simulink subsystem "PvtSubSys_LATC"  (R2020b)
settings: Solver=VariableStepAuto  StartTime=0.0  StopTime=10.0  RelTol=1e-3
values from neighbouring files (symbols this model uses):
  P_Global_CharSpd_ms : value not decoded    [PubParsGlobal.sldd]
  P_Global_SteeringAngleRatio : value not decoded    [PubParsGlobal.sldd]
  P_Global_WheelBase_m : value not decoded    [PubParsGlobal.sldd]
  P_LCS_A0_Dis_BP : value not decoded    [SubMdlDD_LATC.sldd]
  P_LCS_A2_Curve_BP : value not decoded    [SubMdlDD_LATC.sldd]
  P_LCS_A2_LatAcc_BP : value not decoded    [SubMdlDD_LATC.sldd]
  P_LCS_A2_Pretime = 0.075    [SubMdlDD_LATC.sldd]
  P_LCS_A2S_FliterTime = 0.5    [SubMdlDD_LATC.sldd]
  P_LCS_AngErrReversSign_SourceSW = 1.0    [SubMdlDD_LATC.sldd]
  P_LCS_AngleErrorReversTorq : value not decoded    [SubMdlDD_LATC.sldd]
  P_LCS_AngleErrorReversTorq_LC_TarAngleBp : value not decoded    [SubMdlDD_LATC.sldd]
  P_LCS_AngleErrorReversTorq_LC_TarAngleFac : value not decoded    [SubMdlDD_LATC.sldd]
  P_LCS_AngleErrorReversTorq_LC_VehSpdBp : value not decoded    [SubMdlDD_LATC.sldd]
  P_LCS_AngleErrorReversTorq_LC_VehSpdVal : value not decoded    [SubMdlDD_LATC.sldd]
  P_LCS_AngleErrorReversTorq_VehSpdBp : value not decoded    [SubMdlDD_LATC.sldd]
  P_LCS_AngleErrorReversTorq_VehSpdFac : value not decoded    [SubMdlDD_LATC.sldd]
  P_LCS_AngleFilterTime = 0.1    [SubMdlDD_LATC.sldd]
  P_LCS_AngleSlope_AES_Active = 0.4 0.4 0.4 0.35 0.35 0.35 0.35 0.35 0.35 0.3 0.3 0.3 0.3 0.3 0.3 0.3 0.3 0.3 0.3 0.4 0.4 0.4 0.35 0.35 0.35 0.35 0.35 0.35 0.3 0.3 0.3 0.3 0.3 0.3 0.3 0.3 0.3 0.3 0.4 0.4 0.4 0.35 0.35 0.35 0.35 0.35 0.35 0.3 0.3 0.3 0.3 0.3 0.3 0.3 0.3 0.3 0.3 0.4 0.4 0.4 0.35 0.35 0.35 0.35 0.35 0.35 0.3 0.3 0.3 0.3 0.3 0.3 0.3 0.3 0.3 0.3 0.4 0.4 0.4 0.35 0.35 0.35 0.35 0.35 0.35 0.3 0.3 0.3 0.3 0.3 0.3 0.3 0.    [SubMdlDD_LATC.sldd]
  P_LCS_AngleSlope_ESS_Add = 1.0 1.0 1.0 1.0 2.0 2.0 2.0 7.0 7.0 7.0 7.0 7.0 7.0 7.0 7.0 7.0 7.0 7.0 7.0 1.0 1.0 1.0 1.0 2.0 2.0 2.0 7.0 7.0 7.0 7.0 7.0 7.0 7.0 7.0 7.0 7.0 7.0 7.0 1.0 1.0 1.0 1.0 2.0 2.0 2.0 7.0 7.0 7.0 7.0 7.0 7.0 7.0 7.0 7.0 7.0 7.0 7.0 1.0 1.0 1.0 1.0 2.0 2.0 2.0 7.0 7.0 7.0 7.0 7.0 7.0 7.0 7.0 7.0 7.0 7.0 7.0 1.0 1.0 1.0 1.0 7.5 7.5 7.5 7.5 7.5 7.5 7.5 7.5 7.5 7.5 7.5 8.0 8.0 8.0 8.0 1.0 1.0 1.0 1.0 7.5    [SubMdlDD_LATC.sldd]
  P_LCS_AngleSlope_LC_Eco = 0.4 0.4 0.4 0.35 0.35 0.35 0.35 0.35 0.35 0.3 0.3 0.3 0.3 0.3 0.3 0.3 0.3 0.3 0.3 0.4 0.4 0.4 0.35 0.35 0.35 0.35 0.35 0.35 0.3 0.3 0.3 0.3 0.3 0.3 0.3 0.3 0.3 0.3 0.4 0.4 0.4 0.35 0.35 0.35 0.35 0.35 0.35 0.3 0.3 0.3 0.3 0.3 0.3 0.3 0.3 0.3 0.3 0.4 0.4 0.4 0.35 0.35 0.35 0.35 0.35 0.35 0.3 0.3 0.3 0.3 0.3 0.3 0.3 0.3 0.3 0.3 0.4 0.4 0.4 0.35 0.35 0.35 0.35 0.35 0.35 0.3 0.3 0.3 0.3 0.3 0.3 0.3 0.    [SubMdlDD_LATC.sldd]
  P_LCS_AngleSlope_LC_Nomal = 0.4 0.4 0.4 0.35 0.35 0.35 0.35 0.35 0.35 0.3 0.3 0.3 0.3 0.3 0.3 0.3 0.3 0.3 0.3 0.4 0.4 0.4 0.35 0.35 0.35 0.35 0.35 0.35 0.3 0.3 0.3 0.3 0.3 0.3 0.3 0.3 0.3 0.3 0.4 0.4 0.4 0.35 0.35 0.35 0.35 0.35 0.35 0.3 0.3 0.3 0.3 0.3 0.3 0.3 0.3 0.3 0.3 0.4 0.4 0.4 0.35 0.35 0.35 0.35 0.35 0.35 0.3 0.3 0.3 0.3 0.3 0.3 0.3 0.3 0.3 0.3 0.4 0.4 0.4 0.35 0.35 0.35 0.35 0.35 0.35 0.3 0.3 0.3 0.3 0.3 0.3 0.3 0.    [SubMdlDD_LATC.sldd]
  P_LCS_AngleSlope_LC_Sport = 0.4 0.4 0.4 0.35 0.35 0.35 0.35 0.35 0.35 0.3 0.3 0.3 0.3 0.3 0.3 0.3 0.3 0.3 0.3 0.4 0.4 0.4 0.35 0.35 0.35 0.35 0.35 0.35 0.3 0.3 0.3 0.3 0.3 0.3 0.3 0.3 0.3 0.3 0.4 0.4 0.4 0.35 0.35 0.35 0.35 0.35 0.35 0.3 0.3 0.3 0.3 0.3 0.3 0.3 0.3 0.3 0.3 0.4 0.4 0.4 0.35 0.35 0.35 0.35 0.35 0.35 0.3 0.3 0.3 0.3 0.3 0.3 0.3 0.3 0.3 0.3 0.4 0.4 0.4 0.35 0.35 0.35 0.35 0.35 0.35 0.3 0.3 0.3 0.3 0.3 0.3 0.3 0.    [SubMdlDD_LATC.sldd]
  P_LCS_AngleSlope_LCK = 0.4 0.4 0.4 0.4 0.4 0.4 0.4 0.4 0.4 0.4 0.4 0.4 0.4 0.4 0.4 0.4 0.4 0.4 0.4 0.4 0.4 0.4 0.4 0.4 0.4 0.4 0.4 0.4 0.4 0.4 0.4 0.4 0.4 0.4 0.4 0.4 0.4 0.4 0.4 0.4 0.4 0.4 0.4 0.4 0.4 0.4 0.4 0.4 0.4 0.4 0.4 0.4 0.4 0.4 0.4 0.4 0.4 0.4 0.4 0.4 0.4 0.4 0.4 0.4 0.4 0.4 0.4 0.4 0.4 0.4 0.4 0.4 0.4 0.4 0.4 0.4 0.4 0.4 0.4 0.4 0.4 0.4 0.4 0.4 0.4 0.4 0.4 0.4 0.4 0.4 0.4 0.4 0.4 0.4 0.4 0.4 0.4 0.4 0.4 0.4    [SubMdlDD_LATC.sldd]
  P_LCS_AngleSlope_LCKIE = 0.4 0.4 0.4 0.4 0.4 0.4 0.4 0.4 0.4 0.4 0.4 0.4 0.4 0.4 0.4 0.4 0.4 0.4 0.4 0.4 0.4 0.4 0.4 0.4 0.4 0.4 0.4 0.4 0.4 0.4 0.4 0.4 0.4 0.4 0.4 0.4 0.4 0.4 0.4 0.4 0.4 0.4 0.4 0.4 0.4 0.4 0.4 0.4 0.4 0.4 0.4 0.4 0.4 0.4 0.4 0.4 0.4 0.4 0.4 0.4 0.4 0.4 0.4 0.4 0.4 0.4 0.4 0.4 0.4 0.4 0.4 0.4 0.4 0.4 0.4 0.4 0.4 0.4 0.4 0.4 0.4 0.4 0.4 0.4 0.4 0.4 0.4 0.4 0.4 0.4 0.4 0.4 0.4 0.4 0.4 0.4 0.4 0.4 0.4 0.4    [SubMdlDD_LATC.sldd]
  P_LCS_AngleSlope_LKA = 0.2 0.2 0.3 0.4 0.4 0.4 0.4 0.4 0.4 0.4 0.4 0.4 0.4 0.4 0.4 0.4 0.4 0.4 0.4 0.2 0.2 0.3 0.4 0.4 0.4 0.4 0.4 0.4 0.4 0.4 0.4 0.4 0.4 0.4 0.4 0.4 0.4 0.4 0.2 0.2 0.3 0.4 0.4 0.4 0.4 0.4 0.4 0.4 0.4 0.4 0.4 0.4 0.4 0.4 0.4 0.4 0.4 0.2 0.2 0.3 0.4 0.4 0.4 0.4 0.4 0.4 0.4 0.4 0.4 0.4 0.4 0.4 0.4 0.4 0.4 0.4 0.2 0.2 0.3 0.4 0.4 0.4 0.4 0.4 0.4 0.4 0.4 0.4 0.4 0.4 0.4 0.4 0.4 0.4 0.4 0.2 0.2 0.3 0.4 0.4    [SubMdlDD_LATC.sldd]
  P_LCS_AngleSlope_Spd_BP : value not decoded    [SubMdlDD_LATC.sldd]
  P_LCS_CurAngleFiltEnable = 1    [SubMdlDD_LATC.sldd]
  P_LCS_CurAngleFilterFC = 2.0    [SubMdlDD_LATC.sldd]
  P_LCS_CurentOffset_LimitValue = 0.001    [SubMdlDD_LATC.sldd]
  P_LCS_CurOffset_SterAngleSpd_Enable = 0.0    [SubMdlDD_LATC.sldd]
  P_LCS_CurOffset_SterAngleSpd_LimitValue = 6.0    [SubMdlDD_LATC.sldd]
  P_LCS_CurOffset_VehicleSpd_LimitValue = 7.0    [SubMdlDD_LATC.sldd]
  P_LCS_CurOffsetA2_Enable = 0.0    [SubMdlDD_LATC.sldd]
  P_LCS_CurOffsetA2_FliterTime = 0.2    [SubMdlDD_LATC.sldd]
  P_LCS_DeltaEps_SpdBp : value not decoded    [SubMdlDD_LATC.sldd]
  P_LCS_DeltaEps_TimeVal : value not decoded    [SubMdlDD_LATC.sldd]
  P_LCS_DesAngle_DelaySample : value not decoded    [SubMdlDD_LATC.sldd]
  P_LCS_DetNoOverRide_DrvTrq_TH : value not decoded    [SubMdlDD_LATC.sldd]
  P_LCS_DetOverRide_DrvTrq_TH : value not decoded    [SubMdlDD_LATC.sldd]
  P_LCS_EPSNotActiveSpdValue = 3.0    [SubMdlDD_LATC.sldd]
  P_LCS_ESS_AngleSlope_Limit = 2.9    [SubMdlDD_LATC.sldd]
  P_LCS_ESS_LogicTest_Enable = 1.0    [SubMdlDD_LATC.sldd]
  P_LCS_ESS_MaxTorqSlope : value not decoded    [SubMdlDD_LATC.sldd]
  P_LCS_ESS_NotActiveFlgDelayTime = 0.0    [SubMdlDD_LATC.sldd]
  P_LCS_ESS_NotActiveFlgDelayTimeSW = 0.0    [SubMdlDD_LATC.sldd]
  P_LCS_ESS_SteerAngleErr : value not decoded    [SubMdlDD_LATC.sldd]
  P_LCS_ESS_SteerAngleFilterTime = 0.2    [SubMdlDD_LATC.sldd]
  P_LCS_ESS_TarAngleFilterTime = 0.2    [SubMdlDD_LATC.sldd]
  P_LCS_ESSAngleSW2 = 0.0    [SubMdlDD_LATC.sldd]
  P_LCS_ESSOverrideTime1 = 0.06    [SubMdlDD_LATC.sldd]
  P_LCS_ESSOverrideTime2 = 0.06    [SubMdlDD_LATC.sldd]
  P_LCS_ESSOverrideTime3 = 0.06    [SubMdlDD_LATC.sldd]
  P_LCS_ESSOverrideValue1 = 20.0    [SubMdlDD_LATC.sldd]
  P_LCS_ESSOverrideValue2 = 20.0    [SubMdlDD_LATC.sldd]
  P_LCS_FF_A0_Speed_Factor : value not decoded    [SubMdlDD_LATC.sldd]
  P_LCS_FF_A0_Torq : value not decoded    [SubMdlDD_LATC.sldd]
  P_LCS_FF_EnableSpd = 5.0    [SubMdlDD_LATC.sldd]
  P_LCS_FF_LCRevs_SpdBP : value not decoded    [SubMdlDD_LATC.sldd]
  P_LCS_FF_LCRevs_SpdVal : value not decoded    [SubMdlDD_LATC.sldd]
  P_LCS_FF_LCRevs_TimeBP : value not decoded    [SubMdlDD_LATC.sldd]
  P_LCS_FF_LCRevs_TimeFacVal : value not decoded    [SubMdlDD_LATC.sldd]
  P_LCS_FF_Param_CurveBp : value not decoded    [SubMdlDD_LATC.sldd]
  P_LCS_FF_Param_CurveFac : value not decoded    [SubMdlDD_LATC.sldd]
  P_LCS_FF_Speed_Bp : value not decoded    [SubMdlDD_LATC.sldd]
  P_LCS_FF_Speed_Factor : value not decoded    [SubMdlDD_LATC.sldd]
  P_LCS_FF_TarAngleTorq_Bp : value not decoded    [SubMdlDD_LATC.sldd]
  P_LCS_FF_TarAngleTorq_Factor : value not decoded    [SubMdlDD_LATC.sldd]
  P_LCS_FFW_Torq_AngleBp : value not decoded    [SubMdlDD_LATC.sldd]
  P_LCS_FFW_Torq_SpdBp : value not decoded    [SubMdlDD_LATC.sldd]
  P_LCS_FFW_Torq_V71 : value not decoded    [SubMdlDD_LATC.sldd]
  P_LCS_FFWSwitch : value not decoded    [SubMdlDD_LATC.sldd]
  P_LCS_IN_Offset_Test_SW = 0.0    [SubMdlDD_LATC.sldd]
  P_LCS_IN_Offset_Test_Value = 0.0    [SubMdlDD_LATC.sldd]
  P_LCS_LatAcc2CurveSW = 0.0    [SubMdlDD_LATC.sldd]
  P_LCS_LC_Complete_PreDisFac : value not decoded    [SubMdlDD_LATC.sldd]
  P_LCS_LCK_preDis_Nomal : value not decoded    [SubMdlDD_LATC.sldd]
  P_LCS_MaxTorqSlope : value not decoded    [SubMdlDD_LATC.sldd]
  P_LCS_NoOverRideTime_TH_s : value not decoded    [SubMdlDD_LATC.sldd]
  P_LCS_Offset_FliterTime = 2.0    [SubMdlDD_LATC.sldd]
  P_LCS_OverRideDetect_enable : value not decoded    [SubMdlDD_LATC.sldd]
  P_LCS_OverRideTime_TH_s : value not decoded    [SubMdlDD_LATC.sldd]
  P_LCS_PID_A0_BP : value not decoded    [SubMdlDD_LATC.sldd]
  P_LCS_PID_A0_FF_SW = 0.0    [SubMdlDD_LATC.sldd]
  P_LCS_PID_A0_P : value not decoded    [SubMdlDD_LATC.sldd]
  P_LCS_PID_AngErrFacBp : value not decoded    [SubMdlDD_LATC.sldd]
  P_LCS_PID_AngErrFacBp_P : value not decoded    [SubMdlDD_LATC.sldd]
  P_LCS_PID_AngErrFacVal : value not decoded    [SubMdlDD_LATC.sldd]
  P_LCS_PID_AngErrFacVal_P : value not decoded    [SubMdlDD_LATC.sldd]
  P_LCS_PID_DisableKi_CurveVal = 0.003    [SubMdlDD_LATC.sldd]
  P_LCS_PID_DrvTorqFacBp : value not decoded    [SubMdlDD_LATC.sldd]
  P_LCS_PID_DrvTorqFacVal : value not decoded    [SubMdlDD_LATC.sldd]
  P_LCS_PID_Ki_TarAng_ESS : value not decoded    [SubMdlDD_LATC.sldd]
  P_LCS_PID_Kp_TarAng_ESS : value not decoded    [SubMdlDD_LATC.sldd]
  P_LCS_PID_Kp_TarAng_ESS2 : value not decoded    [SubMdlDD_LATC.sldd]
  P_LCS_PID_Kp_TarTorq_ESS : value not decoded    [SubMdlDD_LATC.sldd]
  P_LCS_PID_Param_CurveBp : value not decoded    [SubMdlDD_LATC.sldd]
  P_LCS_PID_Param_CurveFac : value not decoded    [SubMdlDD_LATC.sldd]
  P_LCS_PID_Param_GainSwitch : value not decoded    [SubMdlDD_LATC.sldd]
  P_LCS_PID_Param_Kd : value not decoded    [SubMdlDD_LATC.sldd]
  P_LCS_PID_Param_KdFilterTime : value not decoded    [SubMdlDD_LATC.sldd]
  P_LCS_PID_Param_Ki : value not decoded    [SubMdlDD_LATC.sldd]
  P_LCS_PID_Param_KiFreaseWhenLC_Enable : value not decoded    [SubMdlDD_LATC.sldd]
  P_LCS_PID_Param_Kp : value not decoded    [SubMdlDD_LATC.sldd]
  P_LCS_PID_Param_Speed_Adapt : value not decoded    [SubMdlDD_LATC.sldd]
  P_LCS_PID_Param_Speed_Factor_D : value not decoded    [SubMdlDD_LATC.sldd]
  P_LCS_PID_Param_Speed_Factor_I : value not decoded    [SubMdlDD_LATC.sldd]
  P_LCS_PID_Param_Speed_Factor_P : value not decoded    [SubMdlDD_LATC.sldd]
  P_LCS_PID_Param_SteerWheelAngle_Adapt : value not decoded    [SubMdlDD_LATC.sldd]
  P_LCS_PID_Param_SteerWheelAngle_Factor_D : value not decoded    [SubMdlDD_LATC.sldd]
  P_LCS_PID_Param_SteerWheelAngle_Factor_P : value not decoded    [SubMdlDD_LATC.sldd]
  P_LCS_PID_Param_SteerWheelSpd_Adapt : value not decoded    [SubMdlDD_LATC.sldd]
  P_LCS_PID_Param_SteerWheelSpd_Factor_D : value not decoded    [SubMdlDD_LATC.sldd]
  P_LCS_PID_Param_SteerWheelSpd_Factor_P : value not decoded    [SubMdlDD_LATC.sldd]
  P_LCS_PID_SteerAngSpdLim : value not decoded    [SubMdlDD_LATC.sldd]
  P_LCS_preDis_AES_Fac = 0.0 0.0 0.0 0.0 -0.1 -0.1 -0.1 -0.1 -0.1 -0.1 0.1 0.1 0.1 0.2 0.2 0.2 0.2 0.2 0.2 0.0 0.0 0.0 0.0 -0.1 -0.1 -0.1 -0.1 -0.1 -0.1 0.1 0.1 0.1 0.2 0.2 0.2 0.2 0.2 0.2 0.0 0.0 0.0 0.0 -0.1 -0.1 -0.1 -0.1 -0.1 -0.1 0.1 0.1 0.1 0.2 0.2 0.2 0.2 0.2 0.2 0.0 0.0 0.0 0.0 -0.1 -0.1 -0.1 -0.1 -0.1 -0.1 0.1 0.1 0.1 0.2 0.2 0.2 0.2 0.2 0.2 0.0 0.0 0.0 0.0 -0.1 -0.1 -0.1 -0.1 -0.1 -0.1 0.2 0.2 0.2 0.35 0.35 0.35    [SubMdlDD_LATC.sldd]
  P_LCS_preDis_LC_Eco_Fac = 0.0 0.0 0.0 0.0 0.25 0.3 0.3 0.3 0.35 0.35 0.45 0.45 0.45 0.55 0.55 0.55 0.55 0.55 0.55 0.0 0.0 0.0 0.0 0.25 0.3 0.3 0.3 0.35 0.35 0.45 0.45 0.45 0.55 0.55 0.55 0.55 0.55 0.55 0.0 0.0 0.0 0.0 0.25 0.3 0.3 0.3 0.35 0.35 0.45 0.45 0.45 0.55 0.55 0.55 0.55 0.55 0.55 0.0 0.0 0.0 0.0 0.25 0.3 0.3 0.3 0.35 0.35 0.45 0.45 0.45 0.55 0.55 0.55 0.55 0.55 0.55 0.0 0.0 0.0 0.0 0.25 0.3 0.3 0.3 0.35 0.35 0.55    [SubMdlDD_LATC.sldd]
  P_LCS_preDis_LC_Fac = 0.0 0.0 0.0 0.0 -0.1 -0.1 -0.1 -0.1 -0.1 -0.1 0.1 0.1 0.1 0.2 0.2 0.2 0.2 0.2 0.2 0.0 0.0 0.0 0.0 -0.1 -0.1 -0.1 -0.1 -0.1 -0.1 0.1 0.1 0.1 0.2 0.2 0.2 0.2 0.2 0.2 0.0 0.0 0.0 0.0 -0.1 -0.1 -0.1 -0.1 -0.1 -0.1 0.1 0.1 0.1 0.2 0.2 0.2 0.2 0.2 0.2 0.0 0.0 0.0 0.0 -0.1 -0.1 -0.1 -0.1 -0.1 -0.1 0.1 0.1 0.1 0.2 0.2 0.2 0.2 0.2 0.2 0.0 0.0 0.0 0.0 -0.1 -0.1 -0.1 -0.1 -0.1 -0.1 0.2 0.2 0.2 0.35 0.35 0.35    [SubMdlDD_LATC.sldd]
  P_LCS_preDis_LC_Nomal_Fac = 0.0 0.0 0.0 0.0 -0.1 -0.1 -0.1 -0.1 -0.1 -0.1 0.1 0.1 0.1 0.2 0.2 0.2 0.2 0.2 0.2 0.0 0.0 0.0 0.0 -0.1 -0.1 -0.1 -0.1 -0.1 -0.1 0.1 0.1 0.1 0.2 0.2 0.2 0.2 0.2 0.2 0.0 0.0 0.0 0.0 -0.1 -0.1 -0.1 -0.1 -0.1 -0.1 0.1 0.1 0.1 0.2 0.2 0.2 0.2 0.2 0.2 0.0 0.0 0.0 0.0 -0.1 -0.1 -0.1 -0.1 -0.1 -0.1 0.1 0.1 0.1 0.2 0.2 0.2 0.2 0.2 0.2 0.0 0.0 0.0 0.0 -0.1 -0.1 -0.1 -0.1 -0.1 -0.1 0.2 0.2 0.2 0.35 0.35 0.35    [SubMdlDD_LATC.sldd]
  P_LCS_preDis_LC_Sport_Fac = 0.0 0.0 0.0 0.0 -0.1 -0.1 -0.1 -0.1 -0.1 -0.1 0.1 0.1 0.1 0.2 0.2 0.2 0.2 0.2 0.2 0.0 0.0 0.0 0.0 -0.1 -0.1 -0.1 -0.1 -0.1 -0.1 0.1 0.1 0.1 0.2 0.2 0.2 0.2 0.2 0.2 0.0 0.0 0.0 0.0 -0.1 -0.1 -0.1 -0.1 -0.1 -0.1 0.1 0.1 0.1 0.2 0.2 0.2 0.2 0.2 0.2 0.0 0.0 0.0 0.0 -0.1 -0.1 -0.1 -0.1 -0.1 -0.1 0.1 0.1 0.1 0.2 0.2 0.2 0.2 0.2 0.2 0.0 0.0 0.0 0.0 -0.1 -0.1 -0.1 -0.1 -0.1 -0.1 0.2 0.2 0.2 0.35 0.35 0.35    [SubMdlDD_LATC.sldd]
  P_LCS_preDis_LCK_A2Curve_Fac2 : value not decoded    [SubMdlDD_LATC.sldd]
  ... (+20 more)
undefined symbols (not defined in the file or in its folder): P_LCS_A2_CurrentOffsetFliterTime, P_LCS_AngleSlope_ELK, P_LCS_AngleSlope_ESS, P_LCS_AngleSlope_LC_Cancel, P_LCS_AngleSlope_LCK_Curve_Fac, P_LCS_CurSteerAngleOffsetLimit_Low, P_LCS_CurSteerAngleOffsetLimit_Up, P_LCS_DesLaneA0, P_LCS_DesLaneA1, P_LCS_ESS_preDis_Nomal, P_LCS_ESSAngleSW, P_LCS_ESSAngSlope_SW, P_LCS_LATC_Effect, P_LCS_MinTorqSlope, P_LCS_PID_Param_Kifactor, P_LCS_preDis_ELK_Fac, P_LCS_preDis_ESS_Fac, P_LCS_preDis_LCK_A2Curve_Fac, P_LCS_preDis_LCK_Fac, P_LCS_StateActiv_AngleSlope, P_LCS_StateActiveFlg_BP, P_LCS_TorqSlope_AngleErrorBp, P_LCS_TorqSlope_AngleErrorVal, P_LCS_TorqSlope_AngleSpdBp, P_LCS_TorqSlope_AngleSpdVal, P_LCS_TorqSlope_TorqErrorBp, P_LCS_TorqSlope_TorqErrorVal
libraries: simulink x59
(part 72 of 75)

== stateflow chart PvtSubSys_LATC/Subsystem/LateralControl/LCS_Angle/Subsystem4/Chart ==
  state LC_FF_Offset [parallel]
    settings: executionOrder=2
    state NoOffset
      applyOffset=false;
    state AddOffset
      en:applyOffset=true;OffsetVal=ff_offsetVal*tarAngleSpdSign;
      du:
      %if tarAngleSpdSign~=tarspdsign
      %   OffsetVal=ff_offsetVal*tarAngleSpdSign;
      %end
    (default) -> NoOffset
    NoOffset -> AddOffset : [flag]
    AddOffset -> NoOffset : [~isLC]
  state LC_ReversFlag [parallel]
    settings: executionOrder=1
    state NoLC
      en:flag=false;sign=desTarSteerAngleSign;revstime=0;
      du:
      if ~isLC && ReversOut
      ReversOut=false;
      end
    state Revers_Sts
      en:flag=true;sign=desTarSteerAngleSign;tarspdsign=tarAngleSpdSign;
      du:revstime=revstime+0.02;
    (default) -> NoLC
    NoLC -> Revers_Sts : [isLC&&isReverse&&(~ReversOut)]
    Revers_Sts -> NoLC : [desTarSteerAngleSign~=sign||tarAngleSpdSign~=tarspdsign]{ReversOut=true;}
  data: isLC input; tarAngleSpdSign input; isReverse input; desTarSteerAngleSign input; flag output; sign local; ReversOut local =false; revstime output =0; tarspdsign local; applyOffset output; ff_offsetVal input; OffsetVal output single =single(0)
